simulink model "PID_Controller_xynew_2018"  (R2018b)
settings: Solver=ode4  StartTime=0.0  StopTime=50  FixedStep=0.01  RelTol=1e-5
InitFcn:
  | % load parameters of the default quadrotor
  | disp('Quadrotor parameters loaded by InitFcn')
  | mdl_quadrotor
undefined symbols (not defined in the file or in its folder): A, B, C, D, pwm, quad
libraries: vrlib x3, realtime_pacer_lib x2, simulink x1
(part 2 of 4)

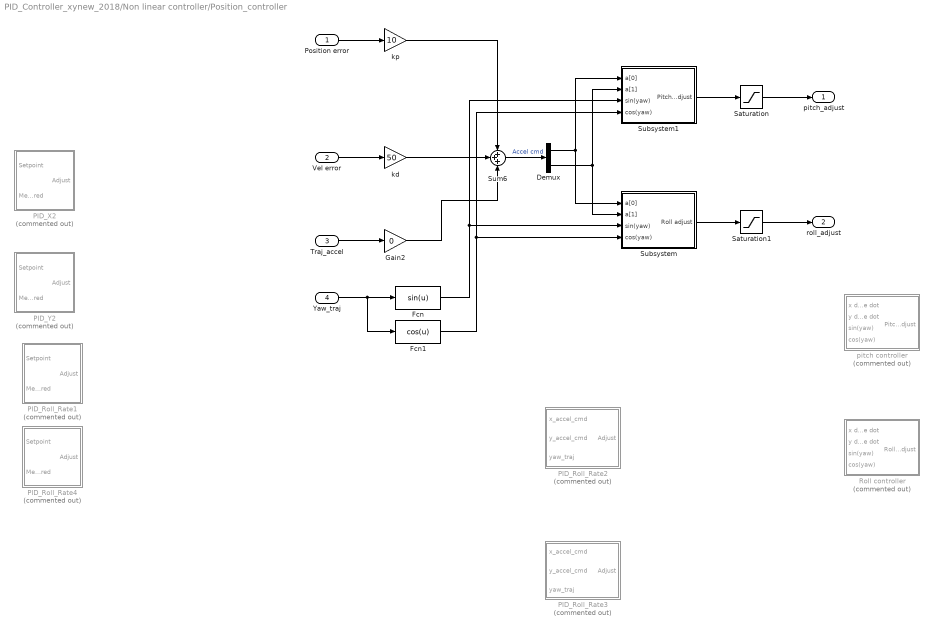
== system PID_Controller_xynew_2018/Non linear controller/Position_controller ==
  Position error : Inport
  Vel error : Inport  Port=2
  Traj_accel : Inport  Port=3
  Yaw_traj : Inport  Port=4
  Demux : Demux  Outputs=2
  Fcn : Fcn  Expr=sin(u)
  Fcn1 : Fcn  Expr=cos(u)
  Gain2 : Gain  Gain=0
  PID_Roll_Rate1 : Subsystem  Commented=on
  PID_Roll_Rate2 : Subsystem  Commented=on
  PID_Roll_Rate3 : Subsystem  Commented=on
  PID_Roll_Rate4 : Subsystem  Commented=on
  PID_X2 : Subsystem  Commented=on
  PID_Y2 : Subsystem  Commented=on
  Roll controller : Subsystem  Commented=on
  Saturation : Saturate  UpperLimit=20  LowerLimit=-20
  Saturation1 : Saturate  UpperLimit=20  LowerLimit=-20
  Subsystem : Subsystem
  Subsystem1 : Subsystem
  Sum6 : Sum  Inputs=+++
  kd : Gain  Gain=50
  kp : Gain  Gain=10
  pitch controller : Subsystem  Commented=on
  pitch_adjust : Outport  VectorParamsAs1DForOutWhenUnconnected=on
  roll_adjust : Outport  Port=2  VectorParamsAs1DForOutWhenUnconnected=on
  wires:
  Position error/1 -> kp/1
  Vel error/1 -> kd/1
  kp/1 -> Sum6/1
  Traj_accel/1 -> Gain2/1
  ? -> PID_Roll_Rate2/3("yaw_traj "), PID_Roll_Rate3/3("yaw_traj ")
  ? -> PID_Roll_Rate2/2(y_accel_cmd), PID_Roll_Rate3/2(y_accel_cmd)
  ? -> PID_Roll_Rate3/1("x_accel_cmd "), PID_Roll_Rate2/1("x_accel_cmd ")
  Sum6/1 -> Demux/1  "Accel cmd"
  Yaw_traj/1 -> Fcn1/1, Fcn/1
  Gain2/1 -> Sum6/3
  Demux/1 -> Subsystem/1(a[0]), Subsystem1/1(a[0])
  Demux/2 -> Subsystem/2(a[1]), Subsystem1/2(a[1])
  Fcn/1 -> Subsystem/3(sin(yaw)), Subsystem1/3(sin(yaw))
  Fcn1/1 -> Subsystem/4(cos(yaw)), Subsystem1/4(cos(yaw))
  Subsystem1/1(Pitch adjust) -> Saturation/1
  Subsystem/1(Roll adjust) -> Saturation1/1
  Saturation/1 -> pitch_adjust/1
  Saturation1/1 -> roll_adjust/1
  kd/1 -> Sum6/2

== system PID_Controller_xynew_2018/Non linear controller/Position_controller1 ==
  X_error : Inport
  Y_error : Inport  Port=2
  dX : Inport  Port=3
  dY : Inport  Port=4
  PID_Roll_Rate2 : Subsystem
  PID_Roll_Rate3 : Subsystem
  PID_X2 : Subsystem
  PID_Y2 : Subsystem
  Saturation : Saturate  UpperLimit=30  LowerLimit=-30
  Saturation1 : Saturate  UpperLimit=30  LowerLimit=-30
  Scope1 : Scope
  Scope2 : Scope
  pitch_adjust : Outport  VectorParamsAs1DForOutWhenUnconnected=on
  roll_adjust : Outport  Port=2  VectorParamsAs1DForOutWhenUnconnected=on
  wires:
  Saturation1/1 -> roll_adjust/1
  PID_Roll_Rate3/1(Adjust) -> Saturation1/1
  Saturation/1 -> pitch_adjust/1, Scope1/1
  PID_Roll_Rate2/1(Adjust) -> Saturation/1, Scope2/1
  dX/1 -> PID_Roll_Rate2/2(Measured)
  X_error/1 -> PID_Roll_Rate2/1(Setpoint)
  dY/1 -> PID_Roll_Rate3/2(Measured)
  Y_error/1 -> PID_Roll_Rate3/1(Setpoint)

== system PID_Controller_xynew_2018/Non linear controller/Position_error ==
  X_cmd : Inport
  Y_cmd : Inport  Port=2
  X : Inport  Port=3
  Y : Inport  Port=4
  "dx, dy " : Inport  Port=5
  "dx, dy cmd" : Inport  Port=6
  Mux : Mux  Inputs=2
  Sum : Sum  Inputs=|+-
  Sum1 : Sum  Inputs=|+-
  Sum2 : Sum  Inputs=|+-
  "Position Error " : Outport  VectorParamsAs1DForOutWhenUnconnected=on
  "Vel Error " : Outport  Port=2  VectorParamsAs1DForOutWhenUnconnected=on
  wires:
  X_cmd/1 -> Sum/1
  X/1 -> Sum/2
  Y_cmd/1 -> Sum1/1
  Y/1 -> Sum1/2
  Sum/1 -> Mux/1
  Sum1/1 -> Mux/2
  "dx, dy cmd"/1 -> Sum2/1
  "dx, dy "/1 -> Sum2/2
  Sum2/1 -> "Vel Error "/1
  Mux/1 -> "Position Error "/1

== system PID_Controller_xynew_2018/Non linear controller/Position_error1 ==
  X_cmd : Inport
  Y_cmd : Inport  Port=2
  X : Inport  Port=3
  Y : Inport  Port=4
  Psi : Inport  Port=5
  Constant1 : Constant  Value=0
  Fcn : Fcn  Expr=sin(u)
  Fcn1 : Fcn  Expr=cos(u)
  Product{,1..3} (4 alike) : Product
  Sum : Sum  Inputs=|+-
  Sum1 : Sum  Inputs=|+-
  Sum2 : Sum  Inputs=|++
  Sum4 : Sum  Inputs=|+-
  X Error in body Frame : Outport  VectorParamsAs1DForOutWhenUnconnected=on
  Y Error in Body Frame : Outport  Port=2  VectorParamsAs1DForOutWhenUnconnected=on
  wires:
  Sum4/1 -> Y Error in Body Frame/1  "Yerr*cos(psi)-Xerr*sin(psi)"
  Product3/1 -> Sum4/2  "Xerr*sin(psi)"
  Sum1/1 -> Product2/1, Product1/1  "Y Error"
  Fcn/1 -> Product3/2, Product2/2  "sin(psi)"
  Sum2/1 -> X Error in body Frame/1  "Xerr*cos(psi)+Yerr*sin(psi)"
  Y_cmd/1 -> Sum1/1
  X_cmd/1 -> Sum/1
  X/1 -> Sum/2
  Y/1 -> Sum1/2
  Sum/1 -> Product3/1, Product/1  "X Error"
  Fcn1/1 -> Product/2, Product1/2  "cos(psi)"
  Product/1 -> Sum2/1  "Xerr*cos(psi)"
  Product2/1 -> Sum2/2  "Yerr*sin(psi)"
  Product1/1 -> Sum4/1  "Yerr*cos(psi)"
  Psi/1 -> Fcn1/1, Fcn/1

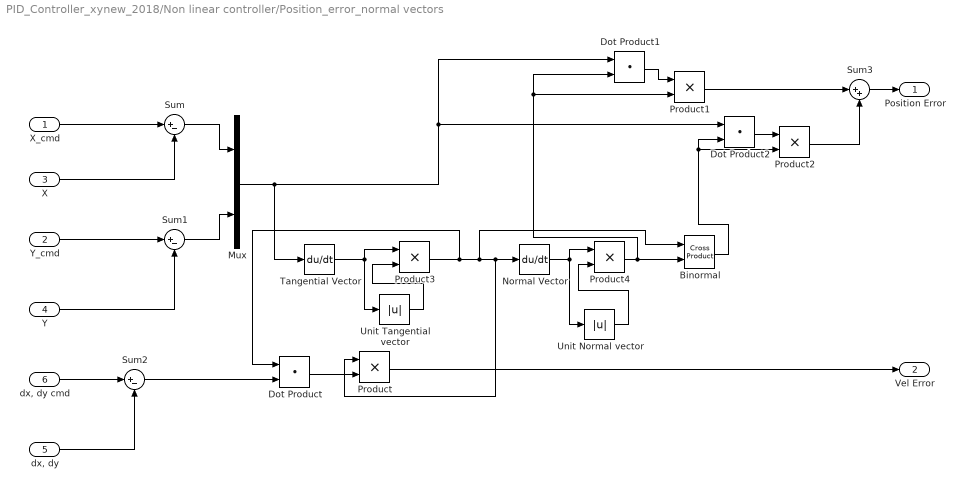
== system PID_Controller_xynew_2018/Non linear controller/Position_error_normal vectors ==
  X_cmd : Inport
  Y_cmd : Inport  Port=2
  X : Inport  Port=3
  Y : Inport  Port=4
  "dx, dy " : Inport  Port=5
  "dx, dy cmd" : Inport  Port=6
  Binormal : vrlib/Utilities/Cross Product
      settings: SourceProductBaseCode=VR
  Dot Product : DotProduct  InputSameDT=on  OutDataTypeStr=Inherit: Inherit via internal rule
  Dot Product1 : DotProduct  InputSameDT=on  OutDataTypeStr=Inherit: Inherit via internal rule
  Dot Product2 : DotProduct  InputSameDT=on  OutDataTypeStr=Inherit: Inherit via internal rule
  Mux : Mux  Inputs=2
  Normal Vector : Derivative
  Product{,1..4} (5 alike) : Product
  Sum : Sum  Inputs=|+-
  Sum1 : Sum  Inputs=|+-
  Sum2 : Sum  Inputs=|+-
  Sum3 : Sum  Inputs=|++
  Tangential Vector : Derivative
  Unit Normal vector : Abs
  Unit Tangential vector : Abs
  "Position Error " : Outport  VectorParamsAs1DForOutWhenUnconnected=on
  "Vel Error " : Outport  Port=2  VectorParamsAs1DForOutWhenUnconnected=on
  wires:
  X_cmd/1 -> Sum/1
  X/1 -> Sum/2
  Y_cmd/1 -> Sum1/1
  Y/1 -> Sum1/2
  Sum/1 -> Mux/1
  Sum1/1 -> Mux/2
  "dx, dy cmd"/1 -> Sum2/1
  "dx, dy "/1 -> Sum2/2
  Sum2/1 -> Dot Product/2
  Tangential Vector/1 -> Product3/1, Unit Tangential vector/1
  Product3/1 -> Dot Product/1, Binormal/1, Product/1, Normal Vector/1
  Normal Vector/1 -> Product4/1, Unit Normal vector/1
  Product/1 -> "Vel Error "/1
  Dot Product/1 -> Product/2
  Product4/1 -> Binormal/2, Product1/2, Dot Product1/2
  Dot Product1/1 -> Product1/1
  Product1/1 -> Sum3/1
  Mux/1 -> Dot Product2/1, Dot Product1/1, Tangential Vector/1
  Binormal/1 -> Product2/2, Dot Product2/2
  Dot Product2/1 -> Product2/1
  Product2/1 -> Sum3/2
  Sum3/1 -> "Position Error "/1
  Unit Tangential vector/1 -> Product3/2
  Unit Normal vector/1 -> Product4/2

== system PID_Controller_xynew_2018/Non linear controller/Rate_controller ==
  dpitch_adjust : Inport
  droll_adjust : Inport  Port=2
  dpitch : Inport  Port=3
  droll : Inport  Port=4
  PID_Pitch_Rate1 : Subsystem
  PID_Pitch_Rate3 : Subsystem
  PID_Roll_Rate1 : Subsystem
  PID_Roll_Rate3 : Subsystem
  pitch_command : Outport  VectorParamsAs1DForOutWhenUnconnected=on
  roll_command : Outport  Port=2  VectorParamsAs1DForOutWhenUnconnected=on
  wires:
  dpitch_adjust/1 -> PID_Roll_Rate3/1(Setpoint)
  PID_Roll_Rate3/1(Adjust) -> pitch_command/1
  droll_adjust/1 -> PID_Roll_Rate1/1(Setpoint)
  droll/1 -> PID_Roll_Rate1/2(Measured)
  PID_Roll_Rate1/1(Adjust) -> roll_command/1
  dpitch/1 -> PID_Roll_Rate3/2(Measured)

== system PID_Controller_xynew_2018/Non linear controller/Yaw_Position_controller ==
  Setpoint : Inport
  Measured : Inport  Port=2
  1/dt : Gain  Gain=1/100  OutMin=[-200]  OutMax=[200]
  Kd : Gain  Gain=0  OutMin=[-200]  OutMax=[200]
  Ki : Gain  Gain=0  OutMin=[-200]  OutMax=[200]
  Kp : Gain  Gain=0.3  OutMin=[-200]  OutMax=[200]
  Memory : Memory
  Memory1 : Memory
  Saturation : Saturate  UpperLimit=166.7  LowerLimit=-166.7
  Sum1 : Sum  Inputs=|++
  Sum2 : Sum  Inputs=|+-
  Sum5 : Sum  Inputs=+++
  Sum6 : Sum  Inputs=+-|
  dt : Gain  Gain=1/100  OutMin=[-200]  OutMax=[200]
  Adjust : Outport  VectorParamsAs1DForOutWhenUnconnected=on
  wires:
  Measured/1 -> Sum6/2  "measured"
  Setpoint/1 -> Sum6/1  "pid_desired"
  Memory/1 -> Sum2/2  "pid_prevError"
  Ki/1 -> Sum5/2
  Sum5/1 -> Adjust/1
  Kp/1 -> Sum5/1
  Kd/1 -> Sum5/3
  dt/1 -> Sum1/1
  Sum2/1 -> 1/dt/1
  1/dt/1 -> Kd/1
  Sum6/1 -> Sum2/1, Memory/1, dt/1, Kp/1  "pid_error"
  Sum1/1 -> Memory1/1, Saturation/1  "pid_integ"
  Memory1/1 -> Sum1/2
  Saturation/1 -> Ki/1

== system PID_Controller_xynew_2018/Non linear controller/Yaw_Rate_controller ==
  Setpoint : Inport
  Measured : Inport  Port=2
  1/dt : Gain  Gain=1/500  OutMin=[-200]  OutMax=[200]
  Kd : Gain  Gain=0  OutMin=[-200]  OutMax=[200]
  Ki : Gain  Gain=16.7  OutMin=[-200]  OutMax=[200]
  Kp : Gain  Gain=70  OutMin=[-200]  OutMax=[200]
  Memory : Memory
  Memory1 : Memory
  Saturation : Saturate  UpperLimit=166.7  LowerLimit=-166.7
  Sum1 : Sum  Inputs=|++
  Sum2 : Sum  Inputs=|+-
  Sum5 : Sum  Inputs=+++
  Sum6 : Sum  Inputs=+-|
  dt : Gain  Gain=1/500  OutMin=[-200]  OutMax=[200]
  Adjust : Outport  VectorParamsAs1DForOutWhenUnconnected=on
  wires:
  Measured/1 -> Sum6/2  "measured"
  Setpoint/1 -> Sum6/1  "pid_desired"
  Memory/1 -> Sum2/2  "pid_prevError"
  Ki/1 -> Sum5/2
  Sum5/1 -> Adjust/1
  Kp/1 -> Sum5/1
  Kd/1 -> Sum5/3
  dt/1 -> Sum1/1
  Sum2/1 -> 1/dt/1
  1/dt/1 -> Kd/1
  Sum6/1 -> Sum2/1, Memory/1, dt/1, Kp/1  "pid_error"
  Sum1/1 -> Memory1/1, Saturation/1  "pid_integ"
  Memory1/1 -> Sum1/2
  Saturation/1 -> Ki/1

== system PID_Controller_xynew_2018/old linear backup/Altitude_controller ==
  Z_in : Inport
  Z : Inport  Port=2
  "Min_thrust " : Constant  Commented=on  Value=pwm  SampleTime=0
  PID_Altitude : Subsystem
  Saturation : Saturate  UpperLimit=60000  LowerLimit=-20000
  Saturation1 : Saturate  UpperLimit=15000  LowerLimit=-20000
  Sum3 : Sum  Inputs=|++
  Base_thrust : Outport  VectorParamsAs1DForOutWhenUnconnected=on
  wires:
  Saturation/1 -> Base_thrust/1
  "Min_thrust "/1 -> Sum3/2
  Sum3/1 -> Saturation/1
  Z/1 -> PID_Altitude/2(Measured)
  Z_in/1 -> PID_Altitude/1(Setpoint)
  Saturation1/1 -> Sum3/1
  PID_Altitude/1(Adjust) -> Saturation1/1

== system PID_Controller_xynew_2018/old linear backup/Attitude_controller ==
  pitch_in : Inport
  roll_in : Inport  Port=2
  pitch : Inport  Port=3
  roll : Inport  Port=4
  PID_Pitch1 : Subsystem
  PID_Pitch3 : Subsystem
  PID_Roll_Rate1 : Subsystem
  PID_Roll_Rate2 : Subsystem
  dpitch_adjust : Outport  VectorParamsAs1DForOutWhenUnconnected=on
  droll_adjust : Outport  Port=2  VectorParamsAs1DForOutWhenUnconnected=on
  wires:
  roll_in/1 -> PID_Roll_Rate1/1(Setpoint)
  roll/1 -> PID_Roll_Rate1/2(Measured)
  PID_Roll_Rate1/1(Adjust) -> droll_adjust/1
  pitch_in/1 -> PID_Roll_Rate2/1(Setpoint)
  pitch/1 -> PID_Roll_Rate2/2(Measured)
  PID_Roll_Rate2/1(Adjust) -> dpitch_adjust/1

== system PID_Controller_xynew_2018/old linear backup/Control_mixer ==
  Pitch : Inport
  "Roll\t" : Inport  Port=2
  Yaw : Inport  Port=3
  T : Inport  Port=4
  Configuration_+ : Subsystem
  Configuration_X1 : Subsystem
  Mode_Selector : Constant  Value=2
  Multiport Switch : MultiPortSwitch  Inputs=2
  Mux : Mux
  Mux1 : Mux
  PWM : Outport  VectorParamsAs1DForOutWhenUnconnected=on
  wires:
  Pitch/1 -> Configuration_X1/1(Pitch), Configuration_+/1(Pitch)
  Configuration_X1/3(W3) -> Mux1/3
  Mux1/1 -> Multiport Switch/3
  Mux/1 -> Multiport Switch/2
  Configuration_X1/4(W4) -> Mux1/4
  T/1 -> Configuration_X1/4(Tau), Configuration_+/4(Tau)
  Multiport Switch/1 -> PWM/1
  Yaw/1 -> Configuration_X1/3(Yaw), Configuration_+/3(Yaw)
  "Roll\t"/1 -> Configuration_X1/2(Roll), Configuration_+/2(Roll)
  Mode_Selector/1 -> Multiport Switch/1
  Configuration_+/2(W2) -> Mux/2
  Configuration_+/1(W1) -> Mux/1
  Configuration_X1/2(W2) -> Mux1/2
  Configuration_X1/1(W1) -> Mux1/1
  Configuration_+/3(W3) -> Mux/3
  Configuration_+/4(W4) -> Mux/4

== system PID_Controller_xynew_2018/old linear backup/Position_controller ==
  Position error : Inport
  Vel error : Inport  Port=2
  Traj_accel : Inport  Port=3
  Yaw_traj : Inport  Port=4
  Demux : Demux  Outputs=2
  Derivative : Derivative  Commented=on
  Fcn : Fcn  Expr=sin(u)
  Fcn1 : Fcn  Expr=cos(u)
  Gain2 : Gain  Gain=0
  PID_Roll_Rate1 : Subsystem  Commented=on
  PID_Roll_Rate2 : Subsystem  Commented=on
  PID_Roll_Rate3 : Subsystem  Commented=on
  PID_Roll_Rate4 : Subsystem  Commented=on
  PID_X2 : Subsystem  Commented=on
  PID_Y2 : Subsystem  Commented=on
  Subsystem : Subsystem
  Subsystem1 : Subsystem
  Sum6 : Sum  Inputs=+++
  kd : Gain  Gain=100
  kp : Gain  Gain=100
  pitch_adjust : Outport  VectorParamsAs1DForOutWhenUnconnected=on
  roll_adjust : Outport  Port=2  VectorParamsAs1DForOutWhenUnconnected=on
  wires:
  Position error/1 -> kp/1
  Vel error/1 -> kd/1
  kp/1 -> Sum6/1
  Traj_accel/1 -> Gain2/1
  ? -> PID_Roll_Rate2/3("yaw_traj "), PID_Roll_Rate3/3("yaw_traj ")
  ? -> PID_Roll_Rate2/2(y_accel_cmd), PID_Roll_Rate3/2(y_accel_cmd)
  ? -> PID_Roll_Rate3/1("x_accel_cmd "), PID_Roll_Rate2/1("x_accel_cmd ")
  Sum6/1 -> Demux/1  "Accel cmd"
  Yaw_traj/1 -> Fcn1/1, Fcn/1
  Gain2/1 -> Sum6/3
  Demux/1 -> Subsystem/1(a[0]), Subsystem1/1(a[0])
  Demux/2 -> Subsystem1/2(a[1]), Subsystem/2(a[1])
  Fcn/1 -> Subsystem1/3(sin(yaw)), Subsystem/3(sin(yaw))
  Fcn1/1 -> Subsystem1/4(cos(yaw)), Subsystem/4(cos(yaw))
  Subsystem/1(Pitch adjust) -> pitch_adjust/1
  Subsystem1/1(Pitch adjust) -> roll_adjust/1
  kd/1 -> Sum6/2

== system PID_Controller_xynew_2018/old linear backup/Position_controller1 ==
  X_error : Inport
  Y_error : Inport  Port=2
  dX : Inport  Port=3
  dY : Inport  Port=4
  PID_Roll_Rate2 : Subsystem
  PID_Roll_Rate3 : Subsystem
  PID_X2 : Subsystem
  PID_Y2 : Subsystem
  Saturation : Saturate  UpperLimit=30  LowerLimit=-30
  Saturation1 : Saturate  UpperLimit=30  LowerLimit=-30
  Scope1 : Scope
  Scope2 : Scope
  pitch_adjust : Outport  VectorParamsAs1DForOutWhenUnconnected=on
  roll_adjust : Outport  Port=2  VectorParamsAs1DForOutWhenUnconnected=on
  wires:
  Saturation1/1 -> roll_adjust/1
  PID_Roll_Rate3/1(Adjust) -> Saturation1/1
  Saturation/1 -> pitch_adjust/1, Scope1/1
  PID_Roll_Rate2/1(Adjust) -> Saturation/1, Scope2/1
  dX/1 -> PID_Roll_Rate2/2(Measured)
  X_error/1 -> PID_Roll_Rate2/1(Setpoint)
  dY/1 -> PID_Roll_Rate3/2(Measured)
  Y_error/1 -> PID_Roll_Rate3/1(Setpoint)

== system PID_Controller_xynew_2018/old linear backup/Position_error ==
  X_cmd : Inport
  Y_cmd : Inport  Port=2
  X : Inport  Port=3
  Y : Inport  Port=4
  "dx, dy " : Inport  Port=5
  "dx, dy cmd" : Inport  Port=6
  Mux : Mux  Inputs=2
  Sum : Sum  Inputs=|+-
  Sum1 : Sum  Inputs=|+-
  Sum2 : Sum  Inputs=|+-
  To Workspace : ToWorkspace  Commented=on  VariableName=traj  SaveFormat=Timeseries  SampleTime=-1
      settings: Decimation=2
  "Position Error " : Outport  VectorParamsAs1DForOutWhenUnconnected=on
  "Vel Error " : Outport  Port=2  VectorParamsAs1DForOutWhenUnconnected=on
  wires:
  X_cmd/1 -> Sum/1
  X/1 -> Sum/2
  Y_cmd/1 -> Sum1/1
  Y/1 -> Sum1/2
  Sum/1 -> Mux/1
  Sum1/1 -> Mux/2
  "dx, dy cmd"/1 -> Sum2/1
  "dx, dy "/1 -> Sum2/2
  Sum2/1 -> "Vel Error "/1
  Mux/1 -> To Workspace/1, "Position Error "/1

== system PID_Controller_xynew_2018/old linear backup/Position_error1 ==
  X_cmd : Inport
  Y_cmd : Inport  Port=2
  X : Inport  Port=3
  Y : Inport  Port=4
  Psi : Inport  Port=5
  Constant1 : Constant  Value=0
  Fcn : Fcn  Expr=sin(u)
  Fcn1 : Fcn  Expr=cos(u)
  Product{,1..3} (4 alike) : Product
  Sum : Sum  Inputs=|+-
  Sum1 : Sum  Inputs=|+-
  Sum2 : Sum  Inputs=|++
  Sum4 : Sum  Inputs=|+-
  X Error in body Frame : Outport  VectorParamsAs1DForOutWhenUnconnected=on
  Y Error in Body Frame : Outport  Port=2  VectorParamsAs1DForOutWhenUnconnected=on
  wires:
  Sum4/1 -> Y Error in Body Frame/1  "Yerr*cos(psi)-Xerr*sin(psi)"
  Product3/1 -> Sum4/2  "Xerr*sin(psi)"
  Sum1/1 -> Product2/1, Product1/1  "Y Error"
  Fcn/1 -> Product3/2, Product2/2  "sin(psi)"
  Sum2/1 -> X Error in body Frame/1  "Xerr*cos(psi)+Yerr*sin(psi)"
  Y_cmd/1 -> Sum1/1
  X_cmd/1 -> Sum/1
  X/1 -> Sum/2
  Y/1 -> Sum1/2
  Sum/1 -> Product3/1, Product/1  "X Error"
  Fcn1/1 -> Product/2, Product1/2  "cos(psi)"
  Product/1 -> Sum2/1  "Xerr*cos(psi)"
  Product2/1 -> Sum2/2  "Yerr*sin(psi)"
  Product1/1 -> Sum4/1  "Yerr*cos(psi)"
  Psi/1 -> Fcn1/1, Fcn/1

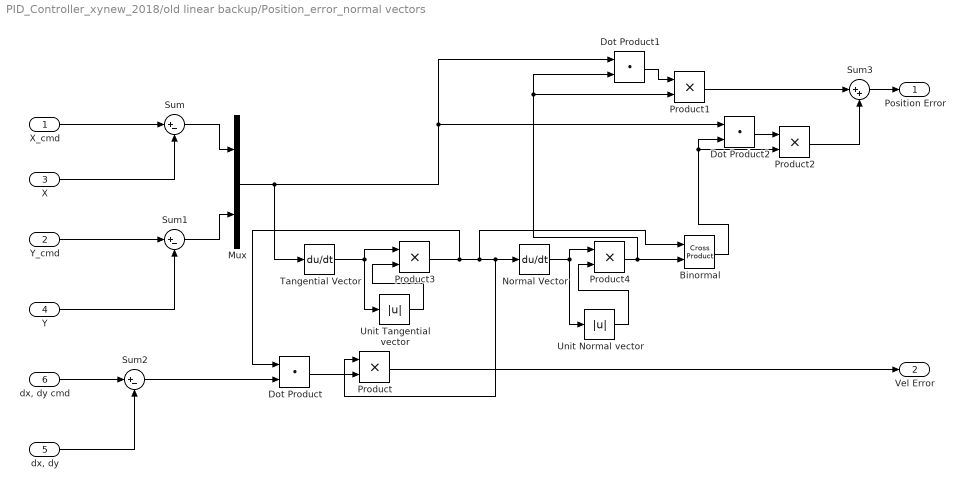
== system PID_Controller_xynew_2018/old linear backup/Position_error_normal vectors ==
  X_cmd : Inport
  Y_cmd : Inport  Port=2
  X : Inport  Port=3
  Y : Inport  Port=4
  "dx, dy " : Inport  Port=5
  "dx, dy cmd" : Inport  Port=6
  Binormal : vrlib/Utilities/Cross Product
      settings: SourceProductBaseCode=VR
  Dot Product : DotProduct  InputSameDT=on  OutDataTypeStr=Inherit: Inherit via internal rule
  Dot Product1 : DotProduct  InputSameDT=on  OutDataTypeStr=Inherit: Inherit via internal rule
  Dot Product2 : DotProduct  InputSameDT=on  OutDataTypeStr=Inherit: Inherit via internal rule
  Mux : Mux  Inputs=2
  Normal Vector : Derivative
  Product{,1..4} (5 alike) : Product
  Sum : Sum  Inputs=|+-
  Sum1 : Sum  Inputs=|+-
  Sum2 : Sum  Inputs=|+-
  Sum3 : Sum  Inputs=|++
  Tangential Vector : Derivative
  Unit Normal vector : Abs
  Unit Tangential vector : Abs
  "Position Error " : Outport  VectorParamsAs1DForOutWhenUnconnected=on
  "Vel Error " : Outport  Port=2  VectorParamsAs1DForOutWhenUnconnected=on
  wires:
  X_cmd/1 -> Sum/1
  X/1 -> Sum/2
  Y_cmd/1 -> Sum1/1
  Y/1 -> Sum1/2
  Sum/1 -> Mux/1
  Sum1/1 -> Mux/2
  "dx, dy cmd"/1 -> Sum2/1
  "dx, dy "/1 -> Sum2/2
  Sum2/1 -> Dot Product/2
  Tangential Vector/1 -> Product3/1, Unit Tangential vector/1
  Product3/1 -> Dot Product/1, Binormal/1, Product/1, Normal Vector/1
  Normal Vector/1 -> Product4/1, Unit Normal vector/1
  Product/1 -> "Vel Error "/1
  Dot Product/1 -> Product/2
  Product4/1 -> Binormal/2, Product1/2, Dot Product1/2
  Dot Product1/1 -> Product1/1
  Product1/1 -> Sum3/1
  Mux/1 -> Dot Product2/1, Dot Product1/1, Tangential Vector/1
  Binormal/1 -> Product2/2, Dot Product2/2
  Dot Product2/1 -> Product2/1
  Product2/1 -> Sum3/2
  Sum3/1 -> "Position Error "/1
  Unit Tangential vector/1 -> Product3/2
  Unit Normal vector/1 -> Product4/2

== system PID_Controller_xynew_2018/old linear backup/Rate_controller ==
  dpitch_adjust : Inport
  droll_adjust : Inport  Port=2
  dpitch : Inport  Port=3
  droll : Inport  Port=4
  PID_Pitch_Rate1 : Subsystem
  PID_Pitch_Rate3 : Subsystem
  PID_Roll_Rate1 : Subsystem
  PID_Roll_Rate3 : Subsystem
  pitch_command : Outport  VectorParamsAs1DForOutWhenUnconnected=on
  roll_command : Outport  Port=2  VectorParamsAs1DForOutWhenUnconnected=on
  wires:
  dpitch_adjust/1 -> PID_Roll_Rate3/1(Setpoint)
  PID_Roll_Rate3/1(Adjust) -> pitch_command/1
  droll_adjust/1 -> PID_Roll_Rate1/1(Setpoint)
  droll/1 -> PID_Roll_Rate1/2(Measured)
  PID_Roll_Rate1/1(Adjust) -> roll_command/1
  dpitch/1 -> PID_Roll_Rate3/2(Measured)

== system PID_Controller_xynew_2018/old linear backup/Yaw_Position_controller ==
  Setpoint : Inport
  Measured : Inport  Port=2
  1/dt : Gain  Gain=1/100  OutMin=[-200]  OutMax=[200]
  Kd : Gain  Gain=0  OutMin=[-200]  OutMax=[200]
  Ki : Gain  Gain=0  OutMin=[-200]  OutMax=[200]
  Kp : Gain  Gain=3  OutMin=[-200]  OutMax=[200]
  Memory : Memory
  Memory1 : Memory
  Saturation : Saturate  UpperLimit=166.7  LowerLimit=-166.7
  Sum1 : Sum  Inputs=|++
  Sum2 : Sum  Inputs=|+-
  Sum5 : Sum  Inputs=+++
  Sum6 : Sum  Inputs=+-|
  dt : Gain  Gain=1/100  OutMin=[-200]  OutMax=[200]
  Adjust : Outport  VectorParamsAs1DForOutWhenUnconnected=on
  wires:
  Measured/1 -> Sum6/2  "measured"
  Setpoint/1 -> Sum6/1  "pid_desired"
  Memory/1 -> Sum2/2  "pid_prevError"
  Ki/1 -> Sum5/2
  Sum5/1 -> Adjust/1
  Kp/1 -> Sum5/1
  Kd/1 -> Sum5/3
  dt/1 -> Sum1/1
  Sum2/1 -> 1/dt/1
  1/dt/1 -> Kd/1
  Sum6/1 -> Sum2/1, Memory/1, dt/1, Kp/1  "pid_error"
  Sum1/1 -> Memory1/1, Saturation/1  "pid_integ"
  Memory1/1 -> Sum1/2
  Saturation/1 -> Ki/1

== system PID_Controller_xynew_2018/old linear backup/Yaw_Rate_controller ==
  Setpoint : Inport
  Measured : Inport  Port=2
  1/dt : Gain  Gain=1/500  OutMin=[-200]  OutMax=[200]
  Kd : Gain  Gain=0  OutMin=[-200]  OutMax=[200]
  Ki : Gain  Gain=16.7  OutMin=[-200]  OutMax=[200]
  Kp : Gain  Gain=70  OutMin=[-200]  OutMax=[200]
  Memory : Memory
  Memory1 : Memory
  Saturation : Saturate  UpperLimit=166.7  LowerLimit=-166.7
  Sum1 : Sum  Inputs=|++
  Sum2 : Sum  Inputs=|+-
  Sum5 : Sum  Inputs=+++
  Sum6 : Sum  Inputs=+-|
  dt : Gain  Gain=1/500  OutMin=[-200]  OutMax=[200]
  Adjust : Outport  VectorParamsAs1DForOutWhenUnconnected=on
  wires:
  Measured/1 -> Sum6/2  "measured"
  Setpoint/1 -> Sum6/1  "pid_desired"
  Memory/1 -> Sum2/2  "pid_prevError"
  Ki/1 -> Sum5/2
  Sum5/1 -> Adjust/1
  Kp/1 -> Sum5/1
  Kd/1 -> Sum5/3
  dt/1 -> Sum1/1
  Sum2/1 -> 1/dt/1
  1/dt/1 -> Kd/1
  Sum6/1 -> Sum2/1, Memory/1, dt/1, Kp/1  "pid_error"
  Sum1/1 -> Memory1/1, Saturation/1  "pid_integ"
  Memory1/1 -> Sum1/2
  Saturation/1 -> Ki/1

== system PID_Controller_xynew_2018/Canada Nonlinear Controller/Altitude_controller/PID_Altitude ==
  Setpoint : Inport
  Measured : Inport  Port=2
  Derivative : Derivative
  Integrator Limited : Integrator  LimitOutput=on  UpperSaturationLimit=1000  LowerSaturationLimit=-1000
  Kd : Gain  Gain=9000  OutMin=[-200]  OutMax=[200]
  Ki : Gain  Gain=3500  OutMin=[-200]  OutMax=[200]
  Kp : Gain  Gain=11000  OutMin=[-200]  OutMax=[200]
  Sum5 : Sum  Inputs=+++
  Sum6 : Sum  Inputs=+-|
  Adjust : Outport  VectorParamsAs1DForOutWhenUnconnected=on
  wires:
  Derivative/1 -> Kd/1
  Integrator Limited/1 -> Ki/1
  Sum6/1 -> Kp/1, Integrator Limited/1, Derivative/1  "pid_error"
  Kd/1 -> Sum5/3
  Kp/1 -> Sum5/1
  Ki/1 -> Sum5/2
  Setpoint/1 -> Sum6/1  "pid_desired"
  Measured/1 -> Sum6/2  "measured"
  Sum5/1 -> Adjust/1

== system PID_Controller_xynew_2018/Canada Nonlinear Controller/Attitude_controller/PID_Pitch1 ==
  Setpoint : Inport
  Measured : Inport  Port=2
  1/dt : Gain  Gain=250  OutMin=[-200]  OutMax=[200]
  Kd : Gain  Gain=0  OutMin=[-200]  OutMax=[200]
  Ki : Gain  Gain=0  OutMin=[-200]  OutMax=[200]
  Kp : Gain  Gain=3.5  OutMin=[-200]  OutMax=[200]
  Memory : Memory
  Memory1 : Memory
  Saturation : Saturate  UpperLimit=20  LowerLimit=-20
  Sum1 : Sum  Inputs=|++
  Sum2 : Sum  Inputs=|+-
  Sum5 : Sum  Inputs=+++
  Sum6 : Sum  Inputs=+-|
  dt : Gain  Gain=1/250  OutMin=[-200]  OutMax=[200]
  Adjust : Outport  VectorParamsAs1DForOutWhenUnconnected=on
  wires:
  Saturation/1 -> Ki/1
  Memory1/1 -> Sum1/2
  Sum1/1 -> Saturation/1, Memory1/1  "pid_integ"
  Sum6/1 -> Kp/1, dt/1, Memory/1, Sum2/1  "pid_error"
  1/dt/1 -> Kd/1
  Sum2/1 -> 1/dt/1
  dt/1 -> Sum1/1
  Kd/1 -> Sum5/3
  Kp/1 -> Sum5/1
  Sum5/1 -> Adjust/1
  Ki/1 -> Sum5/2
  Memory/1 -> Sum2/2  "pid_prevError"
  Setpoint/1 -> Sum6/1  "pid_desired"
  Measured/1 -> Sum6/2  "measured"

== system PID_Controller_xynew_2018/Canada Nonlinear Controller/Attitude_controller/PID_Pitch3 ==
  Setpoint : Inport
  Measured : Inport  Port=2
  1/dt : Gain  Gain=250  OutMin=[-200]  OutMax=[200]
  Kd : Gain  Gain=0  OutMin=[-200]  OutMax=[200]
  Ki : Gain  Gain=0  OutMin=[-200]  OutMax=[200]
  Kp : Gain  Gain=3.5  OutMin=[-200]  OutMax=[200]
  Memory : Memory
  Memory1 : Memory
  Saturation : Saturate  UpperLimit=20  LowerLimit=-20
  Sum1 : Sum  Inputs=|++
  Sum2 : Sum  Inputs=|+-
  Sum5 : Sum  Inputs=+++
  Sum6 : Sum  Inputs=+-|
  dt : Gain  Gain=1/250  OutMin=[-200]  OutMax=[200]
  Adjust : Outport  VectorParamsAs1DForOutWhenUnconnected=on
  wires:
  Measured/1 -> Sum6/2  "measured"
  Setpoint/1 -> Sum6/1  "pid_desired"
  Memory/1 -> Sum2/2  "pid_prevError"
  Ki/1 -> Sum5/2
  Sum5/1 -> Adjust/1
  Kp/1 -> Sum5/1
  Kd/1 -> Sum5/3
  dt/1 -> Sum1/1
  Sum2/1 -> 1/dt/1
  1/dt/1 -> Kd/1
  Sum6/1 -> Sum2/1, Memory/1, dt/1, Kp/1  "pid_error"
  Sum1/1 -> Memory1/1, Saturation/1  "pid_integ"
  Memory1/1 -> Sum1/2
  Saturation/1 -> Ki/1

== system PID_Controller_xynew_2018/Canada Nonlinear Controller/Attitude_controller/PID_Roll_Rate1 ==
  Setpoint : Inport
  Measured : Inport  Port=2
  Derivative : Derivative
  Integrator Limited : Integrator  LimitOutput=on  UpperSaturationLimit=20  LowerSaturationLimit=-20
  Kd : Gain  Gain=0  OutMin=[-200]  OutMax=[200]
  Ki : Gain  Gain=2  OutMin=[-200]  OutMax=[200]
  Kp : Gain  Gain=3.5  OutMin=[-200]  OutMax=[200]
  Scope : Scope
  Sum5 : Sum  Inputs=+++
  Sum6 : Sum  Inputs=+-|
  Adjust : Outport  VectorParamsAs1DForOutWhenUnconnected=on
  wires:
  Measured/1 -> Sum6/2  "measured"
  Setpoint/1 -> Sum6/1  "pid_desired"
  Ki/1 -> Sum5/2
  Sum5/1 -> Adjust/1
  Kp/1 -> Sum5/1
  Kd/1 -> Sum5/3
  Sum6/1 -> Derivative/1, Integrator Limited/1, Kp/1  "pid_error"
  Integrator Limited/1 -> Scope/1, Ki/1
  Derivative/1 -> Kd/1

== system PID_Controller_xynew_2018/Canada Nonlinear Controller/Attitude_controller/PID_Roll_Rate2 ==
  Setpoint : Inport
  Measured : Inport  Port=2
  Derivative : Derivative
  Integrator Limited : Integrator  LimitOutput=on  UpperSaturationLimit=20  LowerSaturationLimit=-20
  Kd : Gain  Gain=0  OutMin=[-200]  OutMax=[200]
  Ki : Gain  Gain=2  OutMin=[-200]  OutMax=[200]
  Kp : Gain  Gain=3.5  OutMin=[-200]  OutMax=[200]
  Scope : Scope
  Sum5 : Sum  Inputs=+++
  Sum6 : Sum  Inputs=+-|
  Adjust : Outport  VectorParamsAs1DForOutWhenUnconnected=on
  wires:
  Derivative/1 -> Kd/1
  Integrator Limited/1 -> Ki/1, Scope/1
  Sum6/1 -> Kp/1, Integrator Limited/1, Derivative/1  "pid_error"
  Kd/1 -> Sum5/3
  Kp/1 -> Sum5/1
  Sum5/1 -> Adjust/1
  Ki/1 -> Sum5/2
  Setpoint/1 -> Sum6/1  "pid_desired"
  Measured/1 -> Sum6/2  "measured"

== system PID_Controller_xynew_2018/Canada Nonlinear Controller/Control_mixer/Configuration_+ ==
  Pitch : Inport
  Roll : Inport  Port=2
  Yaw : Inport  Port=3
  Tau : Inport  Port=4
  Sum{1,9..12} (5 alike) : Sum  Inputs=|++  SaturateOnIntegerOverflow=on  InputSameDT=on  OutDataTypeStr=Inherit: Same as first input
  Sum3 : Sum  Inputs=|--  SaturateOnIntegerOverflow=on  InputSameDT=on  OutDataTypeStr=Inherit: Same as first input
  Sum5 : Sum  Inputs=|-+  SaturateOnIntegerOverflow=on  InputSameDT=on  OutDataTypeStr=Inherit: Same as first input
  Sum7 : Sum  Inputs=|+-  SaturateOnIntegerOverflow=on  InputSameDT=on  OutDataTypeStr=Inherit: Same as first input
  W1 : Outport  VectorParamsAs1DForOutWhenUnconnected=on
  W2 : Outport  Port=2  VectorParamsAs1DForOutWhenUnconnected=on
  W3 : Outport  Port=3  VectorParamsAs1DForOutWhenUnconnected=on
  W4 : Outport  Port=4  VectorParamsAs1DForOutWhenUnconnected=on
  wires:
  Sum5/1 -> Sum11/1
  Yaw/1 -> Sum7/2, Sum5/2, Sum3/2, Sum1/2
  Tau/1 -> Sum11/2, Sum12/2, Sum10/2, Sum9/2
  Sum9/1 -> W1/1
  Pitch/1 -> Sum1/1, Sum5/1
  Roll/1 -> Sum3/1, Sum7/1
  Sum11/1 -> W3/1
  Sum12/1 -> W4/1
  Sum7/1 -> Sum12/1
  Sum10/1 -> W2/1
  Sum1/1 -> Sum9/1
  Sum3/1 -> Sum10/1

== system PID_Controller_xynew_2018/Canada Nonlinear Controller/Control_mixer/Configuration_X1 ==
  Pitch : Inport
  Roll : Inport  Port=2
  Yaw : Inport  Port=3
  Tau : Inport  Port=4
  Gain : Gain  Gain=0.5
  Gain1 : Gain  Gain=0.5
  Sum1 : Sum  Inputs=|+-+  SaturateOnIntegerOverflow=on  InputSameDT=on  OutDataTypeStr=Inherit: Same as first input
  Sum{9..12} (4 alike) : Sum  Inputs=|++  SaturateOnIntegerOverflow=on  InputSameDT=on  OutDataTypeStr=Inherit: Same as first input
  Sum3 : Sum  Inputs=|++-  SaturateOnIntegerOverflow=on  InputSameDT=on  OutDataTypeStr=Inherit: Same as first input
  Sum5 : Sum  Inputs=|+-+  SaturateOnIntegerOverflow=on  InputSameDT=on  OutDataTypeStr=Inherit: Same as first input
  Sum7 : Sum  Inputs=|---  SaturateOnIntegerOverflow=on  InputSameDT=on  OutDataTypeStr=Inherit: Same as first input
  W1 : Outport  VectorParamsAs1DForOutWhenUnconnected=on
  W2 : Outport  Port=2  VectorParamsAs1DForOutWhenUnconnected=on
  W3 : Outport  Port=3  VectorParamsAs1DForOutWhenUnconnected=on
  W4 : Outport  Port=4  VectorParamsAs1DForOutWhenUnconnected=on
  wires:
  Sum3/1 -> Sum11/1
  Yaw/1 -> Sum5/3, Sum3/3, Sum7/3, Sum1/3
  Tau/1 -> Sum11/2, Sum12/2, Sum10/2, Sum9/2
  Sum5/1 -> Sum12/1
  Sum7/1 -> Sum9/1
  Sum1/1 -> Sum10/1
  Roll/1 -> Gain1/1
  Pitch/1 -> Gain/1
  Gain/1 -> Sum7/1, Sum1/1, Sum5/2, Sum3/2
  Gain1/1 -> Sum7/2, Sum1/2, Sum5/1, Sum3/1
  Sum9/1 -> W1/1
  Sum10/1 -> W2/1
  Sum11/1 -> W3/1
  Sum12/1 -> W4/1

== system PID_Controller_xynew_2018/Canada Nonlinear Controller/Position_controller/PID_Roll_Rate2 ==
  Setpoint : Inport
  Measured : Inport  Port=2
  Derivative : Derivative
  Integrator Limited : Integrator  LimitOutput=on  UpperSaturationLimit=0.1  LowerSaturationLimit=-0.1
  Kd : Gain  Gain=0  OutMin=[-200]  OutMax=[200]
  Ki : Gain  Gain=2  OutMin=[-200]  OutMax=[200]
  Kp : Gain  Gain=30  OutMin=[-200]  OutMax=[200]
  Scope : Scope
  Sum5 : Sum  Inputs=+++
  Sum6 : Sum  Inputs=+-|
  Adjust : Outport  VectorParamsAs1DForOutWhenUnconnected=on
  wires:
  Measured/1 -> Sum6/2  "measured"
  Setpoint/1 -> Sum6/1  "pid_desired"
  Ki/1 -> Sum5/2
  Sum5/1 -> Adjust/1
  Kp/1 -> Sum5/1
  Kd/1 -> Sum5/3
  Sum6/1 -> Derivative/1, Integrator Limited/1, Kp/1  "pid_error"
  Integrator Limited/1 -> Scope/1, Ki/1
  Derivative/1 -> Kd/1

== system PID_Controller_xynew_2018/Canada Nonlinear Controller/Position_controller/PID_Roll_Rate3 ==
  Setpoint : Inport
  Measured : Inport  Port=2
  Derivative : Derivative
  Integrator Limited : Integrator  LimitOutput=on  UpperSaturationLimit=0.1  LowerSaturationLimit=-0.1
  Kd : Gain  Gain=0  OutMin=[-200]  OutMax=[200]
  Ki : Gain  Gain=-2  OutMin=[-200]  OutMax=[200]
  Kp : Gain  Gain=-30  OutMin=[-200]  OutMax=[200]
  Scope : Scope
  Sum5 : Sum  Inputs=+++
  Sum6 : Sum  Inputs=+-|
  Adjust : Outport  VectorParamsAs1DForOutWhenUnconnected=on
  wires:
  Derivative/1 -> Kd/1
  Integrator Limited/1 -> Ki/1, Scope/1
  Sum6/1 -> Kp/1, Integrator Limited/1, Derivative/1  "pid_error"
  Kd/1 -> Sum5/3
  Kp/1 -> Sum5/1
  Sum5/1 -> Adjust/1
  Ki/1 -> Sum5/2
  Setpoint/1 -> Sum6/1  "pid_desired"
  Measured/1 -> Sum6/2  "measured"

== system PID_Controller_xynew_2018/Canada Nonlinear Controller/Position_controller/PID_X2 ==
  Setpoint : Inport
  Measured : Inport  Port=2
  1/dt : Gain  Gain=100  OutMin=[-200]  OutMax=[200]
  Kd : Gain  Gain=0  OutMin=[-200]  OutMax=[200]
  Ki : Gain  OutMin=[-200]  OutMax=[200]
  Kp : Gain  Gain=15  OutMin=[-200]  OutMax=[200]
  Memory : Memory
  Memory1 : Memory
  Saturation : Saturate  UpperLimit=0.1  LowerLimit=-0.1
  Scope1 : Scope
  Scope2 : Scope
  Sum1 : Sum  Inputs=|++
  Sum2 : Sum  Inputs=|+-
  Sum5 : Sum  Inputs=+++
  Sum6 : Sum  Inputs=+-|
  dt : Gain  Gain=1/100  OutMin=[-200]  OutMax=[200]
  Adjust : Outport  VectorParamsAs1DForOutWhenUnconnected=on
  wires:
  Measured/1 -> Sum6/2
  Saturation/1 -> Ki/1, Scope2/1
  Memory1/1 -> Sum1/2
  Sum1/1 -> Saturation/1, Scope1/1, Memory1/1  "pid_integ"
  Sum6/1 -> Kp/1, dt/1, Memory/1, Sum2/1  "pid_error"
  1/dt/1 -> Kd/1
  Sum2/1 -> 1/dt/1
  dt/1 -> Sum1/1
  Kd/1 -> Sum5/3
  Kp/1 -> Sum5/1
  Sum5/1 -> Adjust/1
  Ki/1 -> Sum5/2
  Memory/1 -> Sum2/2  "pid_prevError"
  Setpoint/1 -> Sum6/1  "pid_desired"

== system PID_Controller_xynew_2018/Canada Nonlinear Controller/Position_controller/PID_Y2 ==
  Setpoint : Inport
  Measured : Inport  Port=2
  1/dt : Gain  Gain=100  OutMin=[-200]  OutMax=[200]
  Kd : Gain  Gain=0  OutMin=[-200]  OutMax=[200]
  Ki : Gain  Gain=-1  OutMin=[-200]  OutMax=[200]
  Kp : Gain  Gain=-15  OutMin=[-200]  OutMax=[200]
  Memory : Memory
  Memory1 : Memory
  Saturation : Saturate  UpperLimit=0.1  LowerLimit=-0.1
  Scope1 : Scope
  Scope2 : Scope
  Sum1 : Sum  Inputs=|++
  Sum2 : Sum  Inputs=|+-
  Sum5 : Sum  Inputs=+++
  Sum6 : Sum  Inputs=+-|
  dt : Gain  Gain=1/100  OutMin=[-200]  OutMax=[200]
  Adjust : Outport  VectorParamsAs1DForOutWhenUnconnected=on
  wires:
  Measured/1 -> Sum6/2
  Saturation/1 -> Ki/1, Scope2/1
  Memory1/1 -> Sum1/2
  Sum1/1 -> Saturation/1, Scope1/1, Memory1/1  "pid_integ"
  Sum6/1 -> Kp/1, dt/1, Memory/1, Sum2/1  "pid_error"
  1/dt/1 -> Kd/1
  Sum2/1 -> 1/dt/1
  dt/1 -> Sum1/1
  Kd/1 -> Sum5/3
  Kp/1 -> Sum5/1
  Sum5/1 -> Adjust/1
  Ki/1 -> Sum5/2
  Memory/1 -> Sum2/2  "pid_prevError"
  Setpoint/1 -> Sum6/1  "pid_desired"

== system PID_Controller_xynew_2018/Canada Nonlinear Controller/Rate_controller/PID_Pitch_Rate1 ==
  Setpoint : Inport
  Measured : Inport  Port=2
  1/dt : Gain  Gain=500  OutMin=[-200]  OutMax=[200]
  Kd : Gain  Gain=0  OutMin=[-200]  OutMax=[200]
  Ki : Gain  Gain=0  OutMin=[-200]  OutMax=[200]
  Kp : Gain  Gain=70  OutMin=[-200]  OutMax=[200]
  Memory : Memory
  Memory1 : Memory
  Saturation : Saturate  UpperLimit=33  LowerLimit=-33
  Sum1 : Sum  Inputs=|++
  Sum2 : Sum  Inputs=|+-
  Sum5 : Sum  Inputs=+++
  Sum6 : Sum  Inputs=+-|
  dt : Gain  Gain=1/500  OutMin=[-200]  OutMax=[200]
  Adjust : Outport  VectorParamsAs1DForOutWhenUnconnected=on
  wires:
  Saturation/1 -> Ki/1
  Memory1/1 -> Sum1/2
  Sum1/1 -> Memory1/1, Saturation/1  "pid_integ"
  Sum6/1 -> Kp/1, dt/1, Memory/1, Sum2/1  "pid_error"
  1/dt/1 -> Kd/1
  Sum2/1 -> 1/dt/1
  dt/1 -> Sum1/1
  Kd/1 -> Sum5/3
  Kp/1 -> Sum5/1
  Sum5/1 -> Adjust/1
  Ki/1 -> Sum5/2
  Memory/1 -> Sum2/2  "pid_prevError"
  Setpoint/1 -> Sum6/1  "pid_desired"
  Measured/1 -> Sum6/2  "measured"

== system PID_Controller_xynew_2018/Canada Nonlinear Controller/Rate_controller/PID_Pitch_Rate3 ==
  Setpoint : Inport
  Measured : Inport  Port=2
  1/dt : Gain  Gain=500  OutMin=[-200]  OutMax=[200]
  Kd : Gain  Gain=0  OutMin=[-200]  OutMax=[200]
  Ki : Gain  Gain=0  OutMin=[-200]  OutMax=[200]
  Kp : Gain  Gain=70  OutMin=[-200]  OutMax=[200]
  Memory : Memory
  Memory1 : Memory
  Saturation : Saturate  UpperLimit=33  LowerLimit=-33
  Sum1 : Sum  Inputs=|++
  Sum2 : Sum  Inputs=|+-
  Sum5 : Sum  Inputs=+++
  Sum6 : Sum  Inputs=+-|
  dt : Gain  Gain=1/500  OutMin=[-200]  OutMax=[200]
  Adjust : Outport  VectorParamsAs1DForOutWhenUnconnected=on
  wires:
  Measured/1 -> Sum6/2  "measured"
  Setpoint/1 -> Sum6/1  "pid_desired"
  Memory/1 -> Sum2/2  "pid_prevError"
  Ki/1 -> Sum5/2
  Sum5/1 -> Adjust/1
  Kp/1 -> Sum5/1
  Kd/1 -> Sum5/3
  dt/1 -> Sum1/1
  Sum2/1 -> 1/dt/1
  1/dt/1 -> Kd/1
  Sum6/1 -> Sum2/1, Memory/1, dt/1, Kp/1  "pid_error"
  Sum1/1 -> Saturation/1, Memory1/1  "pid_integ"
  Memory1/1 -> Sum1/2
  Saturation/1 -> Ki/1

== system PID_Controller_xynew_2018/Canada Nonlinear Controller/Rate_controller/PID_Roll_Rate1 ==
  Setpoint : Inport
  Measured : Inport  Port=2
  Derivative : Derivative
  Integrator Limited : Integrator  LimitOutput=on  UpperSaturationLimit=1000  LowerSaturationLimit=-1000
  Kd : Gain  Gain=0  OutMin=[-200]  OutMax=[200]
  Ki : Gain  Gain=0  OutMin=[-200]  OutMax=[200]
  Kp : Gain  Gain=70  OutMin=[-200]  OutMax=[200]
  Scope : Scope
  Sum5 : Sum  Inputs=+++
  Sum6 : Sum  Inputs=+-|
  Adjust : Outport  VectorParamsAs1DForOutWhenUnconnected=on
  wires:
  Measured/1 -> Sum6/2  "measured"
  Setpoint/1 -> Sum6/1  "pid_desired"
  Ki/1 -> Sum5/2
  Sum5/1 -> Adjust/1
  Kp/1 -> Sum5/1
  Kd/1 -> Sum5/3
  Sum6/1 -> Derivative/1, Integrator Limited/1, Kp/1  "pid_error"
  Integrator Limited/1 -> Scope/1, Ki/1
  Derivative/1 -> Kd/1

== system PID_Controller_xynew_2018/Canada Nonlinear Controller/Rate_controller/PID_Roll_Rate3 ==
  Setpoint : Inport
  Measured : Inport  Port=2
  Derivative : Derivative
  Integrator Limited : Integrator  LimitOutput=on  UpperSaturationLimit=1000  LowerSaturationLimit=-1000
  Kd : Gain  Gain=0  OutMin=[-200]  OutMax=[200]
  Ki : Gain  Gain=0  OutMin=[-200]  OutMax=[200]
  Kp : Gain  Gain=70  OutMin=[-200]  OutMax=[200]
  Scope : Scope
  Sum5 : Sum  Inputs=+++
  Sum6 : Sum  Inputs=+-|
  Adjust : Outport  VectorParamsAs1DForOutWhenUnconnected=on
  wires:
  Derivative/1 -> Kd/1
  Integrator Limited/1 -> Ki/1, Scope/1
  Sum6/1 -> Kp/1, Integrator Limited/1, Derivative/1  "pid_error"
  Kd/1 -> Sum5/3
  Kp/1 -> Sum5/1
  Sum5/1 -> Adjust/1
  Ki/1 -> Sum5/2
  Setpoint/1 -> Sum6/1  "pid_desired"
  Measured/1 -> Sum6/2  "measured"

== system PID_Controller_xynew_2018/Linear Controller/Altitude_controller/PID_Altitude ==
  Setpoint : Inport
  Measured : Inport  Port=2
  Derivative : Derivative
  Integrator Limited : Integrator  LimitOutput=on  UpperSaturationLimit=1000  LowerSaturationLimit=-1000
  Kd : Gain  Gain=9000  OutMin=[-200]  OutMax=[200]
  Ki : Gain  Gain=3500  OutMin=[-200]  OutMax=[200]
  Kp : Gain  Gain=11000  OutMin=[-200]  OutMax=[200]
  Sum5 : Sum  Inputs=+++
  Sum6 : Sum  Inputs=+-|
  Adjust : Outport  VectorParamsAs1DForOutWhenUnconnected=on
  wires:
  Derivative/1 -> Kd/1
  Integrator Limited/1 -> Ki/1
  Sum6/1 -> Kp/1, Integrator Limited/1, Derivative/1  "pid_error"
  Kd/1 -> Sum5/3
  Kp/1 -> Sum5/1
  Ki/1 -> Sum5/2
  Setpoint/1 -> Sum6/1  "pid_desired"
  Measured/1 -> Sum6/2  "measured"
  Sum5/1 -> Adjust/1

== system PID_Controller_xynew_2018/Linear Controller/Attitude_controller/PID_Pitch1 ==
  Setpoint : Inport
  Measured : Inport  Port=2
  1/dt : Gain  Gain=250  OutMin=[-200]  OutMax=[200]
  Kd : Gain  Gain=0  OutMin=[-200]  OutMax=[200]
  Ki : Gain  Gain=0  OutMin=[-200]  OutMax=[200]
  Kp : Gain  Gain=3.5  OutMin=[-200]  OutMax=[200]
  Memory : Memory
  Memory1 : Memory
  Saturation : Saturate  UpperLimit=20  LowerLimit=-20
  Sum1 : Sum  Inputs=|++
  Sum2 : Sum  Inputs=|+-
  Sum5 : Sum  Inputs=+++
  Sum6 : Sum  Inputs=+-|
  dt : Gain  Gain=1/250  OutMin=[-200]  OutMax=[200]
  Adjust : Outport  VectorParamsAs1DForOutWhenUnconnected=on
  wires:
  Saturation/1 -> Ki/1
  Memory1/1 -> Sum1/2
  Sum1/1 -> Saturation/1, Memory1/1  "pid_integ"
  Sum6/1 -> Kp/1, dt/1, Memory/1, Sum2/1  "pid_error"
  1/dt/1 -> Kd/1
  Sum2/1 -> 1/dt/1
  dt/1 -> Sum1/1
  Kd/1 -> Sum5/3
  Kp/1 -> Sum5/1
  Sum5/1 -> Adjust/1
  Ki/1 -> Sum5/2
  Memory/1 -> Sum2/2  "pid_prevError"
  Setpoint/1 -> Sum6/1  "pid_desired"
  Measured/1 -> Sum6/2  "measured"

== system PID_Controller_xynew_2018/Linear Controller/Attitude_controller/PID_Pitch3 ==
  Setpoint : Inport
  Measured : Inport  Port=2
  1/dt : Gain  Gain=250  OutMin=[-200]  OutMax=[200]
  Kd : Gain  Gain=0  OutMin=[-200]  OutMax=[200]
  Ki : Gain  Gain=0  OutMin=[-200]  OutMax=[200]
  Kp : Gain  Gain=3.5  OutMin=[-200]  OutMax=[200]
  Memory : Memory
  Memory1 : Memory
  Saturation : Saturate  UpperLimit=20  LowerLimit=-20
  Sum1 : Sum  Inputs=|++
  Sum2 : Sum  Inputs=|+-
  Sum5 : Sum  Inputs=+++
  Sum6 : Sum  Inputs=+-|
  dt : Gain  Gain=1/250  OutMin=[-200]  OutMax=[200]
  Adjust : Outport  VectorParamsAs1DForOutWhenUnconnected=on
  wires:
  Measured/1 -> Sum6/2  "measured"
  Setpoint/1 -> Sum6/1  "pid_desired"
  Memory/1 -> Sum2/2  "pid_prevError"
  Ki/1 -> Sum5/2
  Sum5/1 -> Adjust/1
  Kp/1 -> Sum5/1
  Kd/1 -> Sum5/3
  dt/1 -> Sum1/1
  Sum2/1 -> 1/dt/1
  1/dt/1 -> Kd/1
  Sum6/1 -> Sum2/1, Memory/1, dt/1, Kp/1  "pid_error"
  Sum1/1 -> Memory1/1, Saturation/1  "pid_integ"
  Memory1/1 -> Sum1/2
  Saturation/1 -> Ki/1

== system PID_Controller_xynew_2018/Linear Controller/Attitude_controller/PID_Roll_Rate1 ==
  Setpoint : Inport
  Measured : Inport  Port=2
  Derivative : Derivative
  Integrator Limited : Integrator  LimitOutput=on  UpperSaturationLimit=20  LowerSaturationLimit=-20
  Kd : Gain  Gain=0  OutMin=[-200]  OutMax=[200]
  Ki : Gain  Gain=2  OutMin=[-200]  OutMax=[200]
  Kp : Gain  Gain=3.5  OutMin=[-200]  OutMax=[200]
  Scope : Scope
  Sum5 : Sum  Inputs=+++
  Sum6 : Sum  Inputs=+-|
  Adjust : Outport  VectorParamsAs1DForOutWhenUnconnected=on
  wires:
  Measured/1 -> Sum6/2  "measured"
  Setpoint/1 -> Sum6/1  "pid_desired"
  Ki/1 -> Sum5/2
  Sum5/1 -> Adjust/1
  Kp/1 -> Sum5/1
  Kd/1 -> Sum5/3
  Sum6/1 -> Derivative/1, Integrator Limited/1, Kp/1  "pid_error"
  Integrator Limited/1 -> Scope/1, Ki/1
  Derivative/1 -> Kd/1

== system PID_Controller_xynew_2018/Linear Controller/Attitude_controller/PID_Roll_Rate2 ==
  Setpoint : Inport
  Measured : Inport  Port=2
  Derivative : Derivative
  Integrator Limited : Integrator  LimitOutput=on  UpperSaturationLimit=20  LowerSaturationLimit=-20
  Kd : Gain  Gain=0  OutMin=[-200]  OutMax=[200]
  Ki : Gain  Gain=2  OutMin=[-200]  OutMax=[200]
  Kp : Gain  Gain=3.5  OutMin=[-200]  OutMax=[200]
  Scope : Scope
  Sum5 : Sum  Inputs=+++
  Sum6 : Sum  Inputs=+-|
  Adjust : Outport  VectorParamsAs1DForOutWhenUnconnected=on
  wires:
  Derivative/1 -> Kd/1
  Integrator Limited/1 -> Ki/1, Scope/1
  Sum6/1 -> Kp/1, Integrator Limited/1, Derivative/1  "pid_error"
  Kd/1 -> Sum5/3
  Kp/1 -> Sum5/1
  Sum5/1 -> Adjust/1
  Ki/1 -> Sum5/2
  Setpoint/1 -> Sum6/1  "pid_desired"
  Measured/1 -> Sum6/2  "measured"

== system PID_Controller_xynew_2018/Linear Controller/Control_mixer/Configuration_+ ==
  Pitch : Inport
  Roll : Inport  Port=2
  Yaw : Inport  Port=3
  Tau : Inport  Port=4
  Sum{1,9..12} (5 alike) : Sum  Inputs=|++  SaturateOnIntegerOverflow=on  InputSameDT=on  OutDataTypeStr=Inherit: Same as first input
  Sum3 : Sum  Inputs=|--  SaturateOnIntegerOverflow=on  InputSameDT=on  OutDataTypeStr=Inherit: Same as first input
  Sum5 : Sum  Inputs=|-+  SaturateOnIntegerOverflow=on  InputSameDT=on  OutDataTypeStr=Inherit: Same as first input
  Sum7 : Sum  Inputs=|+-  SaturateOnIntegerOverflow=on  InputSameDT=on  OutDataTypeStr=Inherit: Same as first input
  W1 : Outport  VectorParamsAs1DForOutWhenUnconnected=on
  W2 : Outport  Port=2  VectorParamsAs1DForOutWhenUnconnected=on
  W3 : Outport  Port=3  VectorParamsAs1DForOutWhenUnconnected=on
  W4 : Outport  Port=4  VectorParamsAs1DForOutWhenUnconnected=on
  wires:
  Sum5/1 -> Sum11/1
  Yaw/1 -> Sum7/2, Sum5/2, Sum3/2, Sum1/2
  Tau/1 -> Sum11/2, Sum12/2, Sum10/2, Sum9/2
  Sum9/1 -> W1/1
  Pitch/1 -> Sum1/1, Sum5/1
  Roll/1 -> Sum3/1, Sum7/1
  Sum11/1 -> W3/1
  Sum12/1 -> W4/1
  Sum7/1 -> Sum12/1
  Sum10/1 -> W2/1
  Sum1/1 -> Sum9/1
  Sum3/1 -> Sum10/1

== system PID_Controller_xynew_2018/Linear Controller/Control_mixer/Configuration_X1 ==
  Pitch : Inport
  Roll : Inport  Port=2
  Yaw : Inport  Port=3
  Tau : Inport  Port=4
  Gain : Gain  Gain=0.5
  Gain1 : Gain  Gain=0.5
  Sum1 : Sum  Inputs=|+-+  SaturateOnIntegerOverflow=on  InputSameDT=on  OutDataTypeStr=Inherit: Same as first input
  Sum{9..12} (4 alike) : Sum  Inputs=|++  SaturateOnIntegerOverflow=on  InputSameDT=on  OutDataTypeStr=Inherit: Same as first input
  Sum3 : Sum  Inputs=|++-  SaturateOnIntegerOverflow=on  InputSameDT=on  OutDataTypeStr=Inherit: Same as first input
  Sum5 : Sum  Inputs=|+-+  SaturateOnIntegerOverflow=on  InputSameDT=on  OutDataTypeStr=Inherit: Same as first input
  Sum7 : Sum  Inputs=|---  SaturateOnIntegerOverflow=on  InputSameDT=on  OutDataTypeStr=Inherit: Same as first input
  W1 : Outport  VectorParamsAs1DForOutWhenUnconnected=on
  W2 : Outport  Port=2  VectorParamsAs1DForOutWhenUnconnected=on
  W3 : Outport  Port=3  VectorParamsAs1DForOutWhenUnconnected=on
  W4 : Outport  Port=4  VectorParamsAs1DForOutWhenUnconnected=on
  wires:
  Sum3/1 -> Sum11/1
  Yaw/1 -> Sum5/3, Sum3/3, Sum7/3, Sum1/3
  Tau/1 -> Sum11/2, Sum12/2, Sum10/2, Sum9/2
  Sum5/1 -> Sum12/1
  Sum7/1 -> Sum9/1
  Sum1/1 -> Sum10/1
  Roll/1 -> Gain1/1
  Pitch/1 -> Gain/1
  Gain/1 -> Sum7/1, Sum1/1, Sum5/2, Sum3/2
  Gain1/1 -> Sum7/2, Sum1/2, Sum5/1, Sum3/1
  Sum9/1 -> W1/1
  Sum10/1 -> W2/1
  Sum11/1 -> W3/1
  Sum12/1 -> W4/1

== system PID_Controller_xynew_2018/Linear Controller/Position_controller/PID_Roll_Rate1 ==
  Setpoint : Inport
  Measured : Inport  Port=2
  Derivative : Derivative
  Integrator Limited : Integrator  LimitOutput=on  UpperSaturationLimit=0.1  LowerSaturationLimit=-0.1
  Kd : Gain  Gain=0  OutMin=[-200]  OutMax=[200]
  Ki : Gain  Gain=2  OutMin=[-200]  OutMax=[200]
  Kp : Gain  Gain=30  OutMin=[-200]  OutMax=[200]
  Scope : Scope
  Sum5 : Sum  Inputs=+++
  Sum6 : Sum  Inputs=+-|
  Adjust : Outport  VectorParamsAs1DForOutWhenUnconnected=on
  wires:
  Measured/1 -> Sum6/2  "measured"
  Setpoint/1 -> Sum6/1  "pid_desired"
  Ki/1 -> Sum5/2
  Sum5/1 -> Adjust/1
  Kp/1 -> Sum5/1
  Kd/1 -> Sum5/3
  Sum6/1 -> Derivative/1, Integrator Limited/1, Kp/1  "pid_error"
  Integrator Limited/1 -> Scope/1, Ki/1
  Derivative/1 -> Kd/1

== system PID_Controller_xynew_2018/Linear Controller/Position_controller/PID_Roll_Rate2 ==
  "x_accel_cmd " : Inport
  y_accel_cmd : Inport  Port=2
  "yaw_traj " : Inport  Port=3
  "1/g " : Constant  Value=1/9.81
  Fcn : Fcn  Expr=sin(u)
  Fcn1 : Fcn  Expr=cos(u)
  Product : Product
  Product1 : Product
  Product2 : Product
  Sum : Sum  Inputs=|+-
  Adjust : Outport  VectorParamsAs1DForOutWhenUnconnected=on
  wires:
  "1/g "/1 -> Product/1
  "x_accel_cmd "/1 -> Product1/1
  "yaw_traj "/1 -> Fcn1/1, Fcn/1
  Fcn/1 -> Product1/2
  y_accel_cmd/1 -> Product2/1
  Fcn1/1 -> Product2/2
  Product1/1 -> Sum/1
  Product2/1 -> Sum/2
  Sum/1 -> Product/2
  Product/1 -> Adjust/1

== system PID_Controller_xynew_2018/Linear Controller/Position_controller/PID_Roll_Rate3 ==
  "x_accel_cmd " : Inport
  y_accel_cmd : Inport  Port=2
  "yaw_traj " : Inport  Port=3
  "1/g " : Constant  Value=1/9.81
  Fcn : Fcn  Expr=sin(u)
  Fcn1 : Fcn  Expr=cos(u)
  Product : Product
  Product1 : Product
  Product2 : Product
  Sum : Sum  Inputs=|+-
  Adjust : Outport  VectorParamsAs1DForOutWhenUnconnected=on
  wires:
  Product2/1 -> Sum/2
  Fcn1/1 -> Product2/2
  Sum/1 -> Product/2
  "x_accel_cmd "/1 -> Product1/1
  "1/g "/1 -> Product/1
  Product/1 -> Adjust/1
  y_accel_cmd/1 -> Product2/1
  Fcn/1 -> Product1/2
  Product1/1 -> Sum/1
  "yaw_traj "/1 -> Fcn1/1, Fcn/1

== system PID_Controller_xynew_2018/Linear Controller/Position_controller/PID_Roll_Rate4 ==
  Setpoint : Inport
  Measured : Inport  Port=2
  Derivative : Derivative
  Integrator Limited : Integrator  LimitOutput=on  UpperSaturationLimit=0.1  LowerSaturationLimit=-0.1
  Kd : Gain  Gain=0  OutMin=[-200]  OutMax=[200]
  Ki : Gain  Gain=-2  OutMin=[-200]  OutMax=[200]
  Kp : Gain  Gain=-30  OutMin=[-200]  OutMax=[200]
  Scope : Scope
  Sum5 : Sum  Inputs=+++
  Sum6 : Sum  Inputs=+-|
  Adjust : Outport  VectorParamsAs1DForOutWhenUnconnected=on
  wires:
  Derivative/1 -> Kd/1
  Integrator Limited/1 -> Ki/1, Scope/1
  Sum6/1 -> Kp/1, Integrator Limited/1, Derivative/1  "pid_error"
  Kd/1 -> Sum5/3
  Kp/1 -> Sum5/1
  Sum5/1 -> Adjust/1
  Ki/1 -> Sum5/2
  Setpoint/1 -> Sum6/1  "pid_desired"
  Measured/1 -> Sum6/2  "measured"

== system PID_Controller_xynew_2018/Linear Controller/Position_controller/PID_X2 ==
  Setpoint : Inport
  Measured : Inport  Port=2
  1/dt : Gain  Gain=100  OutMin=[-200]  OutMax=[200]
  Kd : Gain  Gain=0  OutMin=[-200]  OutMax=[200]
  Ki : Gain  OutMin=[-200]  OutMax=[200]
  Kp : Gain  Gain=15  OutMin=[-200]  OutMax=[200]
  Memory : Memory
  Memory1 : Memory
  Saturation : Saturate  UpperLimit=0.1  LowerLimit=-0.1
  Scope1 : Scope
  Scope2 : Scope
  Sum1 : Sum  Inputs=|++
  Sum2 : Sum  Inputs=|+-
  Sum5 : Sum  Inputs=+++
  Sum6 : Sum  Inputs=+-|
  dt : Gain  Gain=1/100  OutMin=[-200]  OutMax=[200]
  Adjust : Outport  VectorParamsAs1DForOutWhenUnconnected=on
  wires:
  Measured/1 -> Sum6/2
  Saturation/1 -> Ki/1, Scope2/1
  Memory1/1 -> Sum1/2
  Sum1/1 -> Saturation/1, Scope1/1, Memory1/1  "pid_integ"
  Sum6/1 -> Kp/1, dt/1, Memory/1, Sum2/1  "pid_error"
  1/dt/1 -> Kd/1
  Sum2/1 -> 1/dt/1
  dt/1 -> Sum1/1
  Kd/1 -> Sum5/3
  Kp/1 -> Sum5/1
  Sum5/1 -> Adjust/1
  Ki/1 -> Sum5/2
  Memory/1 -> Sum2/2  "pid_prevError"
  Setpoint/1 -> Sum6/1  "pid_desired"

== system PID_Controller_xynew_2018/Linear Controller/Position_controller/PID_Y2 ==
  Setpoint : Inport
  Measured : Inport  Port=2
  1/dt : Gain  Gain=100  OutMin=[-200]  OutMax=[200]
  Kd : Gain  Gain=0  OutMin=[-200]  OutMax=[200]
  Ki : Gain  Gain=-1  OutMin=[-200]  OutMax=[200]
  Kp : Gain  Gain=-15  OutMin=[-200]  OutMax=[200]
  Memory : Memory
  Memory1 : Memory
  Saturation : Saturate  UpperLimit=0.1  LowerLimit=-0.1
  Scope1 : Scope
  Scope2 : Scope
  Sum1 : Sum  Inputs=|++
  Sum2 : Sum  Inputs=|+-
  Sum5 : Sum  Inputs=+++
  Sum6 : Sum  Inputs=+-|
  dt : Gain  Gain=1/100  OutMin=[-200]  OutMax=[200]
  Adjust : Outport  VectorParamsAs1DForOutWhenUnconnected=on
  wires:
  Measured/1 -> Sum6/2
  Saturation/1 -> Ki/1, Scope2/1
  Memory1/1 -> Sum1/2
  Sum1/1 -> Saturation/1, Scope1/1, Memory1/1  "pid_integ"
  Sum6/1 -> Kp/1, dt/1, Memory/1, Sum2/1  "pid_error"
  1/dt/1 -> Kd/1
  Sum2/1 -> 1/dt/1
  dt/1 -> Sum1/1
  Kd/1 -> Sum5/3
  Kp/1 -> Sum5/1
  Sum5/1 -> Adjust/1
  Ki/1 -> Sum5/2
  Memory/1 -> Sum2/2  "pid_prevError"
  Setpoint/1 -> Sum6/1  "pid_desired"

== system PID_Controller_xynew_2018/Linear Controller/Position_controller/Roll controller ==
  x double dot : Inport
  y double dot : Inport  Port=2
  sin(yaw) : Inport  Port=3
  cos(yaw) : Inport  Port=4
  Fcn1 : Fcn  Expr=1/(u)
  Gain : Gain  Gain=1/9.81
  Product : Product
  Product1 : Product
  Product2 : Product
  Square : Math  Operator=square  SaturateOnIntegerOverflow=on
  Square1 : Math  Operator=square  SaturateOnIntegerOverflow=on
  Sum : Sum  Inputs=|+-
  Sum1 : Sum  Inputs=+-
  Roll adjust : Outport
  wires:
  x double dot/1 -> Product/1
  sin(yaw)/1 -> Product1/2, Square1/1
  Product/1 -> Sum1/1
  cos(yaw)/1 -> Product/2, Square/1
  y double dot/1 -> Product1/1
  Product1/1 -> Sum1/2
  Gain/1 -> Product2/1
  Sum1/1 -> Gain/1
  Square/1 -> Sum/1
  Square1/1 -> Sum/2
  Sum/1 -> Fcn1/1
  Product2/1 -> Roll adjust/1
  Fcn1/1 -> Product2/2

== system PID_Controller_xynew_2018/Linear Controller/Position_controller/Subsystem ==
  a[0] : Inport
  a[1] : Inport  Port=2
  sin(yaw) : Inport  Port=3
  cos(yaw) : Inport  Port=4
  Gain : Gain  Gain=1/9.81
  Product : Product
  Product1 : Product
  Sum1 : Sum  Inputs=+-
  Roll adjust : Outport
  wires:
  a[0]/1 -> Product/1
  sin(yaw)/1 -> Product/2
  Product/1 -> Sum1/1
  cos(yaw)/1 -> Product1/2
  a[1]/1 -> Product1/1
  Product1/1 -> Sum1/2
  Gain/1 -> Roll adjust/1
  Sum1/1 -> Gain/1
